simulink model "ex1_1"  (R2021a)
settings: Solver=VariableStepAuto  StartTime=0.0  StopTime=simTime  MaxStep=calculationPrecision  RelTol=1e-3
values from neighbouring files (symbols this model uses):
  Kp = 1/A_Go_wco    [ex8_2_4_calcul_regulateur_PID.m]
undefined symbols (not defined in the file or in its folder): alpha, delay, g, Ka1, Kmv, m, tSlope, vc
settings Model: Creator=ocean  LastModifiedBy=ocean

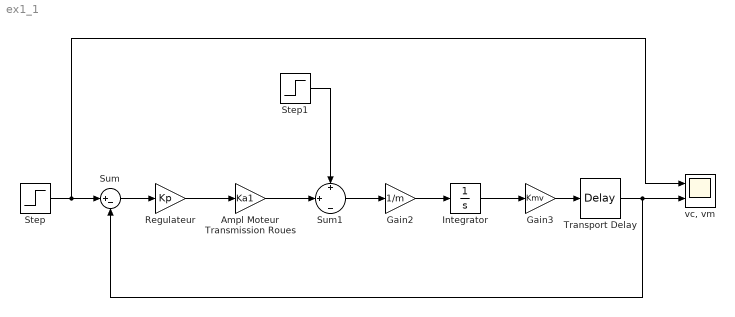
== system ex1_1 ==
  "Ampl Moteur Transmission Roues " : Gain  Gain=Ka1
  Gain2 : Gain  Gain=1/m
  Gain3 : Gain  Gain=Kmv
  Integrator : Integrator
  Regulateur : Gain  Gain=Kp
  Step : Step  After=vc  SampleTime=0
  Step1 : Step  Time=tSlope  After=-m*g*sin(alpha)  SampleTime=0
  Sum : Sum  Inputs=|+-
  Sum1 : Sum  Inputs=+|+|-
  Transport Delay : TransportDelay  DelayTime=delay
  "vc, vm" : Scope  NumInputPorts=2
  wires:
  Regulateur/1 -> "Ampl Moteur Transmission Roues "/1
  Sum/1 -> Regulateur/1
  "Ampl Moteur Transmission Roues "/1 -> Sum1/2
  Sum1/1 -> Gain2/1
  Gain2/1 -> Integrator/1
  Integrator/1 -> Gain3/1
  Gain3/1 -> Transport Delay/1
  Step/1 -> "vc, vm"/1, Sum/1
  Step1/1 -> Sum1/1
  Transport Delay/1 -> Sum/2, "vc, vm"/2
